simulink model "sl_zerotorque"  (R2022a)
settings: Solver=ode45  StartTime=0.0  StopTime=1.5  RelTol=1e-3  EnableMultiTasking=on
PreLoadFcn:
  | if ~exist("ur5", "var")
  |    ur5 = loadrobot("universalUR5e", DataFormat="row", Gravity=[0 0 -9.81]);
  | end
  | 
  | if ~exist("ur5conf", "var")
  |   ur5conf.qn = [0 -1.07 1.38 -0.3 0 -2.3];
  | end
InitFcn:
  | if ~exist("ur5", "var")
  |    ur5 = loadrobot("universalUR5e", DataFormat="row", Gravity=[0 0 -9.81]);
  | end
  | 
  | if ~exist("ur5conf", "var")
  |   ur5conf.qn = [0 -1.07 1.38 -0.3 0 -2.3];
  | end
undefined symbols (not defined in the file or in its folder): conf
libraries: robotmaniplib x1, roblocks x1
Description:
  | Forward dynamics example for UR5 robot collapsing under gravity.
  | 
  | Robotics, Vision and Control - 3rd Edition; Section 9.3
settings Model: ExtModeTrigMode=oneshot  ExtModeArmWhenConnect=off  Creator=pic  LastModifiedBy=rpill
settings SolverCC: AlgebraicLoopSolver=TrustRegion  MaxZcPerStep=1
settings DataIOCC: SaveFormat=Array  SignalLoggingSaveFormat=ModelDataLogs  SignalLogging=off
settings OptimizationCC: BlockReduction=off  BooleanDataType=off  ExpressionDepthLimit=2147483647  InitFltsAndDblsToZero=on  LifeSpan=inf
settings DebuggingCC: SaveWithParameterizedLinksMsg=none  UnderspecifiedInitializationDetection=Classic  MergeDetectMultiDrivingBlocksExec=none  SignalResolutionControl=TryResolveAllWithWarning  MultiTaskDSMMsg=warning  MultiTaskCondExecSysMsg=none  FcnCallInpInsideContextMsg=warning  UnconnectedInputMsg=warning  UnconnectedOutputMsg=warning  UnconnectedLineMsg=warning  AllowSymbolicDim=off  StateNameClashWarn=warning  SFUnexpectedBacktrackingDiag=warning  SFNoUnconditionalDefaultTransitionDiag=warning  SFExecutionAtInitializationDiag=none  SFMachineParentedDataDiag=warning  ArithmeticOperatorsInVariantConditions=warning
settings HardwareCC: ProdBitPerPointer=32  ProdBitPerSizeT=32  ProdBitPerPtrDiffT=32  ProdLargestAtomicFloat=None  ProdIntDivRoundTo=Undefined  ProdEndianess=Unspecified  ProdWordSize=32  ProdHWDeviceType=32-bit Generic  TargetUnknown=on
settings ModelReferenceCC: PropagateSignalLabelsOutOfModel=off
settings SFSimCC: SimUseLocalCustomCode=off  CustomCodeUndefinedFunction=UseInterfaceOnly
settings RTWCC: RTWUseLocalCustomCode=off
settings CodeAppCC: StateflowObjectComments=on
settings GRTTargetCC: TargetLangStandard=C89/C90 (ANSI)  ModelReferenceCompliant=off  ParMdlRefBuildCompliant=off  CompOptLevelCompliant=off  CombineOutputUpdateFcns=off  MatFileLogging=off  GRTInterface=on
settings ConfigComp: CovMetricSettings=dw  CovSaveCumulativeToWorkspaceVar=on  CovSaveSingleToWorkspaceVar=on  CovExternalEMLEnable=off  CovSFcnEnable=off

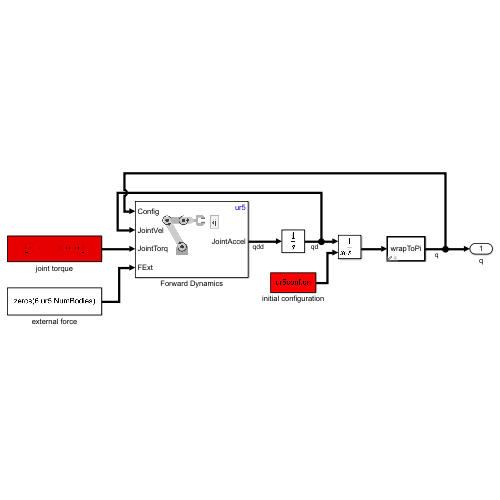
[thumbnail: Simulink's stored preview of the top-level diagram]
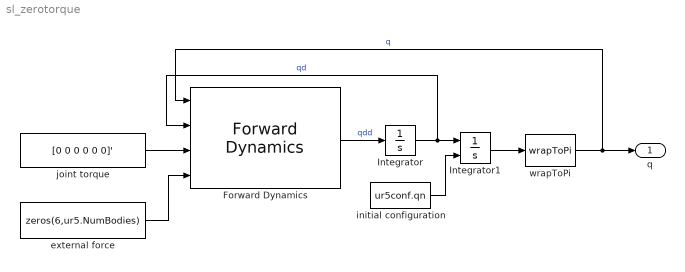
== system sl_zerotorque ==
  Forward Dynamics : robotmaniplib/Forward Dynamics  RigidBodyTree=ur5  SimulateUsing=Interpreted execution
  Integrator : Integrator
  Integrator1 : Integrator  InitialConditionSource=external  InitialCondition=conf.qs
  external force : Constant  Value=zeros(6,ur5.NumBodies)
  initial configuration : Constant  Value=ur5conf.qn
  joint torque : Constant  Value=[0 0 0 0 0 0]'
  wrapToPi : roblocks/wrapToPi
  q : Outport
  wires:
  joint torque/1 -> Forward Dynamics/3
  Integrator/1 -> Integrator1/1, Forward Dynamics/2  "qd"
  external force/1 -> Forward Dynamics/4
  Forward Dynamics/1 -> Integrator/1  "qdd"
  Integrator1/1 -> wrapToPi/1
  wrapToPi/1 -> Forward Dynamics/1, q/1  "q"
  initial configuration/1 -> Integrator1/2
